simulink library "Pump_Simple"  (R2016b)
settings: Solver=ode45  StartTime=0.0  StopTime=10.0  RelTol=1e-3  EnableMultiTasking=on
undefined symbols (not defined in the file): Water
libraries: carnot x1
settings Model: Creator=lena.frank  LastModifiedBy=drhf
settings DataIOCC: LimitDataPoints=on  SaveFormat=Array  SignalLoggingSaveFormat=ModelDataLogs
settings OptimizationCC: ExpressionDepthLimit=2147483647  LifeSpan=inf
settings DebuggingCC: UnderspecifiedInitializationDetection=Classic  MergeDetectMultiDrivingBlocksExec=none  SolverPrmCheckMsg=warning  FcnCallInpInsideContextMsg=warning  StateNameClashWarn=warning  SFUnexpectedBacktrackingDiag=warning  SFNoUnconditionalDefaultTransitionDiag=warning  SFExecutionAtInitializationDiag=none
settings HardwareCC: ProdBitPerPointer=32  ProdBitPerSizeT=32  ProdBitPerPtrDiffT=32  ProdLargestAtomicFloat=None  ProdIntDivRoundTo=Undefined  ProdEndianess=Unspecified  ProdWordSize=32  ProdHWDeviceType=32-bit Generic
settings ModelReferenceCC: PropagateSignalLabelsOutOfModel=off
settings GRTTargetCC: TargetLangStandard=C89/C90 (ANSI)  GeneratePreprocessorConditionals=Disable all  CombineOutputUpdateFcns=off  GRTInterface=on
settings ConfigComp: CovMetricSettings=dw  CovHtmlReporting=on  CovSaveCumulativeToWorkspaceVar=on  CovSaveSingleToWorkspaceVar=on  CovExternalEMLEnable=off

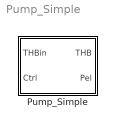
== system Pump_Simple ==
  Pump_Simple : Subsystem  mask(simple Pump){mdotmax=1200/3600, dia=0.025, power=power, fluid_id=Water, mix=0, mix2=0, mix3=0, p0=2e5}
      mask prompts: mdotmax "massflow rate [kg/s]"; dia "diameter at in- and outlet [m]"; power "electric power consumption [W]"; fluid_id "fluid"; mix "fluid mixture 1 [0..1]"; mix2 "fluid mixture 2 [0..1]"; mix3 "fluid mixture 3 [0..1]"; p0 "system pressure [Pa]"
      mask help:
      | Set constant massflow rate according to the control signal.
      | The pump is a very basic model, sometimes creating algebraic loops. If you have problems with algebraic loops, use "Pump_const" instead.
      mask Help: web(fullfile(path_carnot('help'),'Pump_Const.html'),'-helpbrowser')
      mask TypeOptions mdotmax: Pump_basic/mdotmax
      mask TypeOptions dia: Pump_basic/dia
      mask TypeOptions power: Pump_basic/power
      mask TypeOptions fluid_id: Pump_basic/fluid_id
      mask TypeOptions mix: Pump_basic/mix
      mask TypeOptions mix2: Pump_basic/mix2
      mask TypeOptions mix3: Pump_basic/mix3
      mask TypeOptions p0: Pump_basic/p0
      mask Display:
      | plot(0,0,100,100,[40,70,40,30,30,40,60,70,70,60,40],[70,50,30,40,60,70,70,60,40,30,30])
      | % port_label('input',1,'THB')
      | % port_label('input',2,'ctr')
      | % port_label('output',1,'THB')
      | % port_label('output',2,'Pel')

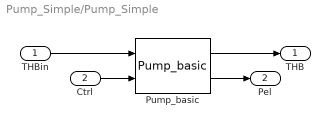
== system Pump_Simple/Pump_Simple ==
  THBin : Inport
  Ctrl : Inport  Port=2
  Pump_basic : carnot/Basic/Hydraulics/Pump_basic  mdotmax=mdotmax  fluid_id=Water  mix=mix  mix2=mix2  mix3=mix3  power=power  p0=p0  dia=dia  ID=No Pressure Drop  hgt=0
  THB : Outport
  Pel : Outport  Port=2
  wires:
  Pump_basic/2 -> Pel/1
  Pump_basic/1 -> THB/1
  Ctrl/1 -> Pump_basic/2
  THBin/1 -> Pump_basic/1
